simulink model "Question_4"  (R2024b)
settings: Solver=VariableStepAuto  StartTime=0.0  StopTime=10.0  RelTol=1e-3
settings Model: Creator=Sagar  LastModifiedBy=Sagar

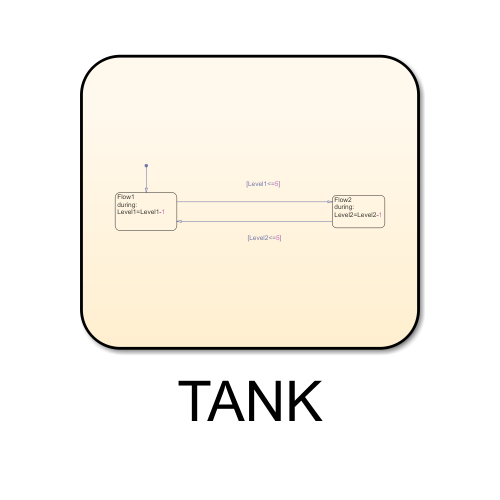
[thumbnail: Simulink's stored preview of the top-level diagram]
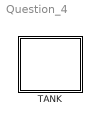
== system Question_4 ==
  TANK : Stateflow chart  TreatAsAtomicUnit=on

== stateflow chart Question_4/TANK ==
  state Flow1
    during:
    Level1=Level1-1
  state Flow2
    during:
    Level2=Level2-1
  (default) -> Flow1
  Flow1 -> Flow2 : [Level1<=5]
  Flow2 -> Flow1 : [Level2<=5]
  data: Level1 local =15; Level2 local =15
